simulink model "monocab"  (R2025a)
settings: Solver=FixedStepDiscrete  StartTime=0.0  StopTime=10.0  FixedStep=1e-4  RelTol=1e-3
undefined symbols (not defined in the file): dspblkCoreblockFVToolHelper, gcbh
libraries: simulink x1
settings Model: Creator=Ismail  LastModifiedBy=Ismail

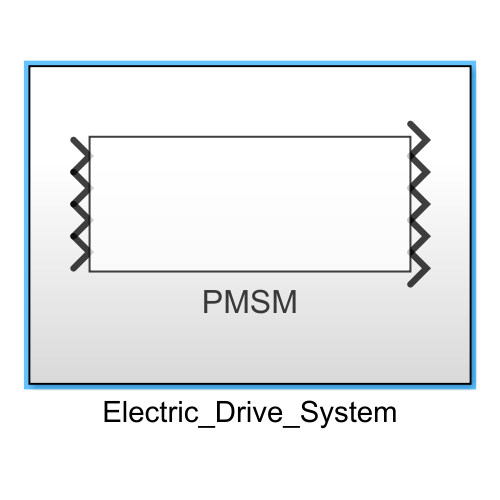
[thumbnail: Simulink's stored preview of the top-level diagram]
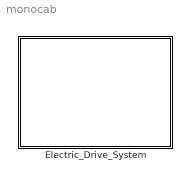
== system monocab ==
  Electric_Drive_System : Subsystem

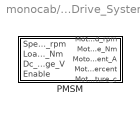
== system monocab/Electric_Drive_System ==
  PMSM : Subsystem

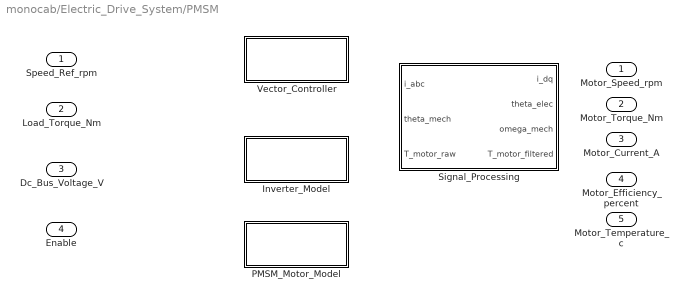
== system monocab/Electric_Drive_System/PMSM ==
  Speed_Ref_rpm : Inport
  Load_Torque_Nm : Inport  Port=2
  Dc_Bus_Voltage_V : Inport  Port=3
  Enable : Inport  Port=4
  Inverter_Model : Subsystem
  PMSM_Motor_Model : Subsystem
  Signal_Processing : Subsystem
  Vector_Controller : Subsystem
  Motor_Speed_rpm : Outport
  Motor_Torque_Nm : Outport  Port=2
  Motor_Current_A : Outport  Port=3
  Motor_Efficiency_percent : Outport  Port=4
  Motor_Temperature_c : Outport  Port=5

== system monocab/Electric_Drive_System/PMSM/Inverter_Model ==

== system monocab/Electric_Drive_System/PMSM/PMSM_Motor_Model ==

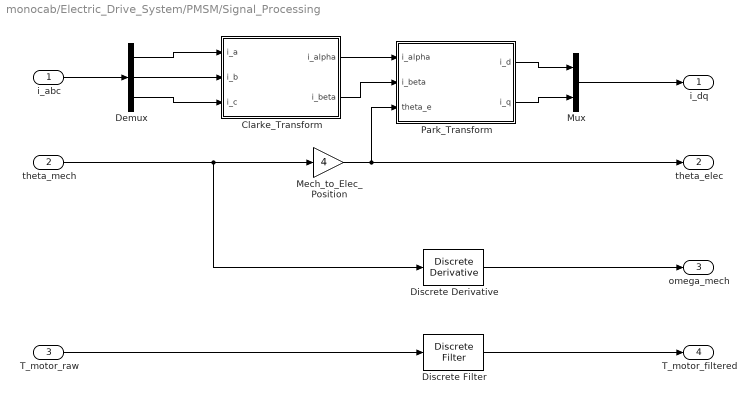
== system monocab/Electric_Drive_System/PMSM/Signal_Processing ==
  i_abc : Inport
  theta_mech : Inport  Port=2
  T_motor_raw : Inport  Port=3
  Clarke_Transform : MATLAB Function  TreatAsAtomicUnit=on
  Demux : Demux  Outputs=3
  Discrete Derivative : simulink/Discrete/Discrete Derivative  gainval=1.0  ICPrevScaledInput=0.0  OutMin=[]  OutMax=[]  OutDataType=fixdt(1, 16)  OutScaling=2^-10  DoSatur=off
  Discrete Filter : DiscreteFilter  LoadFcn=dspblkCoreblockFVToolHelper(gcbh,'load');
      settings: CopyFcn=dspblkCoreblockFVToolHelper(gcbh,'copy');  DeleteFcn=dspblkCoreblockFVToolHelper(gcbh,'close');  ModelCloseFcn=dspblkCoreblockFVToolHelper(gcbh,'close');  PreSaveFcn=dspblkCoreblockFVToolHelper(gcbh,'presave');  PostSaveFcn=dspblkCoreblockFVToolHelper(gcbh,'postsave');  CloseFcn=dspblkCoreblockFVToolHelper(gcbh,'close');
  Mech_to_Elec_Position : Gain  Gain=4
  Mux : Mux  Inputs=2
  Park_Transform : MATLAB Function  TreatAsAtomicUnit=on
  i_dq : Outport
  theta_elec : Outport  Port=2
  omega_mech : Outport  Port=3
  T_motor_filtered : Outport  Port=4
  wires:
  Clarke_Transform/1(i_alpha) -> Park_Transform/1(i_alpha)
  Clarke_Transform/2(i_beta) -> Park_Transform/2(i_beta)
  i_abc/1 -> Demux/1
  Demux/1 -> Clarke_Transform/1(i_a)
  Demux/2 -> Clarke_Transform/2(i_b)
  Demux/3 -> Clarke_Transform/3(i_c)
  Park_Transform/1(i_d) -> Mux/1
  theta_mech/1 -> Discrete Derivative/1, Mech_to_Elec_Position/1
  Mech_to_Elec_Position/1 -> theta_elec/1, Park_Transform/3(theta_e)
  Discrete Derivative/1 -> omega_mech/1
  T_motor_raw/1 -> Discrete Filter/1
  Discrete Filter/1 -> T_motor_filtered/1
  Park_Transform/2(i_q) -> Mux/2
  Mux/1 -> i_dq/1

== system monocab/Electric_Drive_System/PMSM/Vector_Controller ==

== matlab function monocab/Electric_Drive_System/PMSM/Signal_Processing/Park_Transform ==
  data: i_alpha input; i_d output; i_beta input; theta_e input; i_q output
function [i_d, i_q] = fcn(i_alpha, i_beta, theta_e)
%% Park Transformation (αβ to dq)
% Engineering Purpose: Transform to synchronously rotating reference frame
% Why: AC quantities become DC quantities in rotating frame
% Result: Easy to control with PI controllers

% Rotation matrix transformation
cos_theta = cos(theta_e);
sin_theta = sin(theta_e);

% Park transformation equations
i_d = i_alpha * cos_theta + i_beta * sin_theta;    % Direct axis (flux component)
i_q = -i_alpha * sin_theta + i_beta * cos_theta;   % Quadrature axis (torque component)

% Engineering insight:
% i_d controls flux (like DC motor field current)
% i_q controls torque (like DC motor armature current)
end

== matlab function monocab/Electric_Drive_System/PMSM/Signal_Processing/Clarke_Transform ==
  data: i_a input; i_alpha output; i_b input; i_c input; i_beta output
function [i_alpha, i_beta] = fcn(i_a, i_b, i_c)
%% Clarke Transformation (abc to αβ)
% Engineering Purpose: Convert 3-phase balanced system to 2-phase orthogonal system
% Why: Reduces complexity from 3 variables to 2 variables
% Mathematical basis: Power-invariant transformation

% Power-invariant Clarke transformation
i_alpha = (2/3) * (i_a - 0.5*i_b - 0.5*i_c);
i_beta = (2/3) * (sqrt(3)/2) * (i_b - i_c);

% Alternative simplified form (when i_a + i_b + i_c = 0):
% i_alpha = i_a;
% i_beta = (1/sqrt(3)) * (i_b - i_c);
end
